simulink model "pcc_backstepping_model_unaware_full_system_PID"  (R2021b)
settings: Solver=VariableStepAuto  StartTime=0.0  StopTime=60  MaxStep=0.001  RelTol=1e-3
values from neighbouring files (symbols this model uses):
  l = out.l.Data    [animate_pcc.m]    (also in config.m = 0.110*[1;1;1])
  q_eq = [-108; 21.5; -3.4]/180*pi    [config.m]
undefined symbols (not defined in the file or in its folder): mu_p_eq, tol_q_stable
libraries: simulink_extras x4, slpidlib x1
settings Model: PauseTimes=0  Creator=maximilianstoelzle  LastModifiedBy=mstolzle
settings RTWCC: BuildConfiguration=Faster Runs

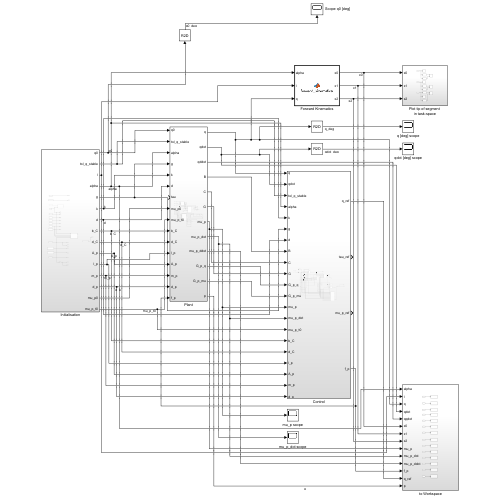
[thumbnail: Simulink's stored preview of the top-level diagram]
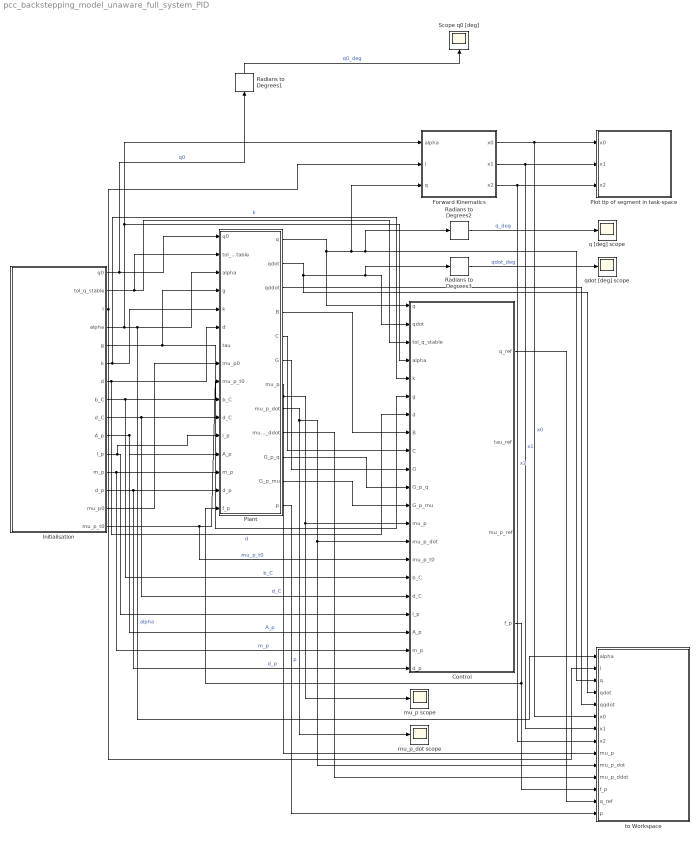
== system pcc_backstepping_model_unaware_full_system_PID ==
  Control : Subsystem
  Forward Kinematics : MATLAB Function  TreatAsAtomicUnit=on
  Initialisation : Subsystem
  Plant : Subsystem
  Plot tip of segment in task-space : Subsystem
  Radians to Degrees1 : simulink_extras/Transformations/Radians to Degrees
  Radians to Degrees2 : simulink_extras/Transformations/Radians to Degrees
  Radians to Degrees3 : simulink_extras/Transformations/Radians to Degrees
  Scope q0 [deg] : Scope
  mu_p scope : Scope
  mu_p_dot scope : Scope
  q [deg] scope : Scope
  qdot [deg] scope : Scope
  to Workspace : Subsystem
  wires:
  Plant/3(qddot) -> to Workspace/5(qqdot)
  Initialisation/12(m_p) -> Plant/14(m_p), Control/20(m_p)  "m_p"
  Initialisation/3(l) -> Forward Kinematics/2(l), to Workspace/2(l)
  Radians to Degrees2/1 -> q [deg] scope/1  "q_deg"
  Initialisation/11(l_p) -> Plant/12(l_p), Control/18(l_p)
  Initialisation/1(q0) -> Radians to Degrees1/1, Plant/1(q0)  "q0"
  Plant/9(mu_p_ddot) -> to Workspace/11(mu_p_ddot)
  Initialisation/14(mu_p0) -> Plant/8(mu_p0)
  Control/1(q_ref) -> to Workspace/13(q_ref)
  Forward Kinematics/3(x2) -> to Workspace/8(x2), Plot tip of segment in task-space/3(x2)  "x2"
  Plant/6(G) -> Control/10(G)
  Plant/11(G_p_mu) -> Control/12(G_p_mu)
  Plant/4(B) -> Control/8(B)
  Initialisation/6(k) -> Control/5(k), Plant/5(k)  "k"
  Radians to Degrees3/1 -> qdot [deg] scope/1  "qdot_deg"
  Radians to Degrees1/1 -> Scope q0 [deg]/1  "q0_deg"
  Initialisation/2(tol_q_stable) -> Plant/2(tol_q_stable), Control/3(tol_q_stable)
  Plant/10(G_p_q) -> Control/11(G_p_q)
  Plant/5(C) -> Control/9(C)
  Initialisation/13(d_p) -> Plant/15(d_p), Control/21(d_p)  "d_p"
  Initialisation/5(g) -> Plant/4(g), Control/6(g)
  Initialisation/4(alpha) -> to Workspace/1(alpha), Plant/3(alpha), Forward Kinematics/1(alpha), Control/4(alpha)  "alpha"
  Initialisation/7(d) -> Plant/6(d), Control/7(d)  "d"
  Plant/2(qdot) -> Control/2(qdot), Radians to Degrees3/1, to Workspace/4(qdot)
  Plant/1(q) -> Radians to Degrees2/1, to Workspace/3(q), Forward Kinematics/3(q), Control/1(q)
  Initialisation/10(A_p) -> Plant/13(A_p), Control/19(A_p)  "A_p"
  Initialisation/9(d_C) -> Plant/11(d_C), Control/17(d_C)  "d_C"
  Initialisation/8(b_C) -> Plant/10(b_C), Control/16(b_C)  "b_C"
  Plant/7(mu_p) -> mu_p scope/1, Control/13(mu_p), to Workspace/9(mu_p)
  Forward Kinematics/1(x0) -> to Workspace/6(x0), Plot tip of segment in task-space/1(x0)  "x0"
  Forward Kinematics/2(x1) -> to Workspace/7(x1), Plot tip of segment in task-space/2(x1)  "x1"
  Control/4(f_p) -> to Workspace/12(f_p), Plant/16(f_p)
  Plant/8(mu_p_dot) -> Control/14(mu_p_dot), to Workspace/10(mu_p_dot), mu_p_dot scope/1
  Initialisation/15(mu_p_t0) -> Control/15(mu_p_t0), Plant/9(mu_p_t0)  "mu_p_t0"
  Plant/12(p) -> to Workspace/14(p)  "p"

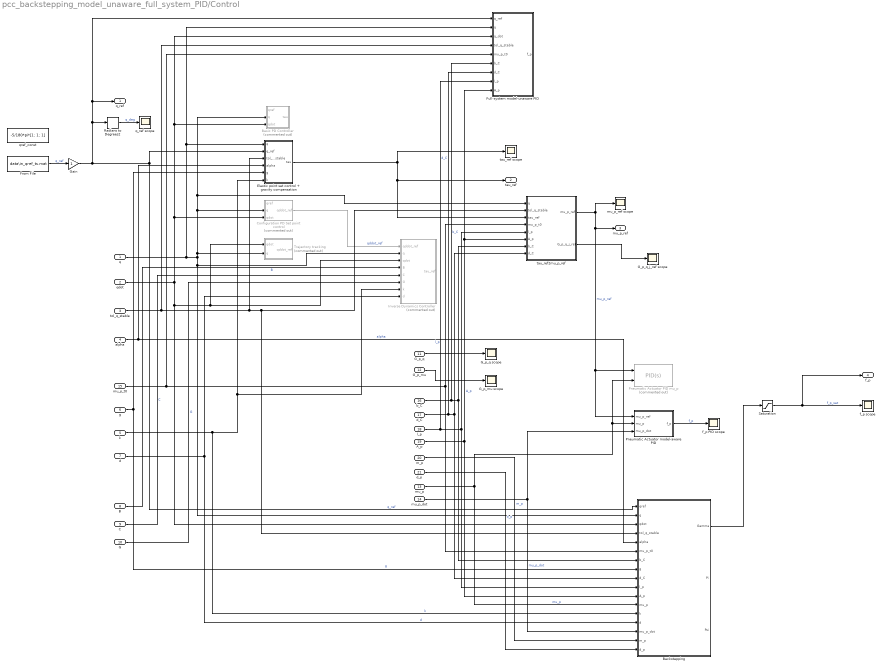
== system pcc_backstepping_model_unaware_full_system_PID/Control ==
  q : Inport
  qdot : Inport  Port=2
  tol_q_stable : Inport  Port=3
  alpha : Inport  Port=4
  k : Inport  Port=5
  g : Inport  Port=6
  d : Inport  Port=7
  B : Inport  Port=8
  C : Inport  Port=9
  G : Inport  Port=10
  G_p_q : Inport  Port=11
  G_p_mu : Inport  Port=12
  mu_p : Inport  Port=13
  mu_p_dot : Inport  Port=14
  mu_p_t0 : Inport  Port=15
  b_C : Inport  Port=16
  d_C : Inport  Port=17
  l_p : Inport  Port=18
  A_p : Inport  Port=19
  m_p : Inport  Port=20
  d_p : Inport  Port=21
  Backstepping : Subsystem
  Basic PD Controller : Subsystem  Commented=on
  Configuration PD Set point control : Subsystem  Commented=on
  Elastic point set control + gravity compensation : MATLAB Function  TreatAsAtomicUnit=on
  From File : FromFile  FileName=data\in_qref_ts.mat  SampleTime=0  InterpolationWithinTimeRange=Zero order hold
  Full-system model-unaware PID : Subsystem
  G_p_mu scope : Scope
  G_p_q scope : Scope
  G_p_q_j_ref scope : Scope
  Gain : Gain
  Inverse Dynamics Controller : MATLAB Function  Commented=on  TreatAsAtomicUnit=on
  Pneumatic Actuator PID mu_p : slpidlib/PID Controller (2DOF)  Commented=on  Controller=PID  Form=Parallel  TimeDomain=Continuous-time  UseExternalTs=off  SampleTime=-1  IntegratorMethod=Forward Euler  FilterMethod=Forward Euler  ControllerParametersSource=internal  P=-3000  I=-500  D=-100  UseFilter=on  N=100  b=1  c=1  TunerSelectOption=Frequency Response Based  InitialConditionSource=internal  InitialConditionForIntegrator=0  InitialConditionForFilter=0  DifferentiatorICPrevScaledInput=0  ExternalReset=none  TrackingMode=off  Kt=1  LimitOutput=off  SatLimitsSource=internal  UpperSaturationLimit=inf  LowerSaturationLimit=-inf  LinearizeAsGain=on  AntiWindupMode=none  Kb=1  POutMin=[]  POutMax=[]  IOutMin=[]  IOutMax=[]  DOutMin=[]  DOutMax=[]  NOutMin=[]  NOutMax=[]  bOutMin=[]  bOutMax=[]  cOutMin=[]  cOutMax=[]  SumOutMin=[]  SumOutMax=[]  SaturationOutMin=[]  SaturationOutMax=[]  PParamMin=[]  PParamMax=[]  IParamMin=[]  IParamMax=[]  DParamMin=[]  DParamMax=[]  NParamMin=[]  NParamMax=[]  bParamMin=[]  bParamMax=[]  cParamMin=[]  cParamMax=[]  KbParamMin=[]  KbParamMax=[]  KtParamMin=[]  KtParamMax=[]  KbOutMin=[]  KbOutMax=[]  KtOutMin=[]  KtOutMax=[]  IntegratorOutMin=[]  IntegratorOutMax=[]  FilterOutMin=[]  FilterOutMax=[]  SumI1OutMin=[]  SumI1OutMax=[]  SumI2OutMin=[]  SumI2OutMax=[]  SumI3OutMin=[]  SumI3OutMax=[]  SumI4OutMin=[]  SumI4OutMax=[]  SumDOutMin=[]  SumDOutMax=[]  Sum1OutMin=[]  Sum1OutMax=[]  Sum2OutMin=[]  Sum2OutMax=[]  Sum3OutMin=[]  Sum3OutMax=[]  DifferentiatorOutMin=[]  DifferentiatorOutMax=[]  FilterDiffOutCoefMin=[]  FilterDiffOutCoefMax=[]  ReciprocalOutMin=[]  ReciprocalOutMax=[]  SumDenOutMin=[]  SumDenOutMax=[]  SumNumOutMin=[]  SumNumOutMax=[]  DivideOutMin=[]  DivideOutMax=[]  UdiffTsProdOutMin=[]  UdiffTsProdOutMax=[]  NTsProdOutMin=[]  NTsProdOutMax=[]  UintegralTsProdOutMin=[]  UintegralTsProdOutMax=[]  UngainTsProdOutMin=[]  UngainTsProdOutMax=[]  IntegratorContinuousStateAttributes=''  IntegratorStateMustResolveToSignalObject=off  IntegratorRTWStateStorageClass=Auto  FilterContinuousStateAttributes=''  FilterStateMustResolveToSignalObject=off  FilterRTWStateStorageClass=Auto  ParallelPVariant=InternalParameters  IdealPVariant=Disabled  IVariant=InternalParameters  DVariant=InternalParameters  bVariant=InternalParameters  cVariant=InternalParameters  IntegratorVariant=Continuous  SatVariant=Disabled  AWVariant=Passthrough  PCopyVariant=Disabled  TRVariant=Disabled  FdbkBlocksVariant=Forward  IdealPFdbkVariant=Disabled  SatFdbkVariant=Disabled  DerivativeFilterVariant=ContFilter  NVariant=InternalParameters  NCopyVariant=Disabled  FilterICVariant=InternalICsFilter  IntegratorICVariant=InternalICs  ExternalResetVariant=Disabled  TRSumVariant=Passthrough  SumFdbkVariant=Disabled  SumVariant=Sum_PID  TsampFilterVariant=InternalTs  TsampNgainVariant=Passthrough  TsampIntegralVariant=Passthrough  ExternalSaturationOutDataTypeStr=Inherit: Same as second input
      settings: SourceProductBaseCode=SL
  Pneumatic Actuator model-aware PID : Subsystem
  Radians to Degrees2 : simulink_extras/Transformations/Radians to Degrees
  Saturation : Saturate  UpperLimit=1000  LowerLimit=-1000
  Trajectory tracking : Subsystem  Commented=on
  f_p PID scope : Scope
  f_p scope : Scope
  mu_p_ref scope : Scope
  q_ref scope : Scope
  qref_const : Constant  Value=-5/180*pi*[1; 1; 1]
  tau_ref scope : Scope
  tau_ref2mu_p_ref : MATLAB Function  TreatAsAtomicUnit=on
  q_ref : Outport
  tau_ref : Outport  Port=2
  mu_p_ref : Outport  Port=3
  f_p : Outport  Port=4
  wires:
  q/1 -> Full-system model-unaware PID/2(q), Elastic point set control + gravity compensation/1(q), Backstepping/2(q), Inverse Dynamics Controller/2(q), Trajectory tracking/2(q), Configuration PD Set point control/2(q), tau_ref2mu_p_ref/1(q), Basic PD Controller/2(q)
  qdot/1 -> Backstepping/3(qdot), Trajectory tracking/1(qdot), Inverse Dynamics Controller/3(qdot), Full-system model-unaware PID/3(q_dot), Basic PD Controller/3(qdot), Configuration PD Set point control/3(qdot)
  B/1 -> Inverse Dynamics Controller/4(B)  "B"
  C/1 -> Inverse Dynamics Controller/5(C)  "C"
  G/1 -> Inverse Dynamics Controller/6(G)  "G"
  k/1 -> Backstepping/13(k), Elastic point set control + gravity compensation/6(k), Inverse Dynamics Controller/7(k)  "k"
  d/1 -> Inverse Dynamics Controller/8(d), Backstepping/14(d)  "d"
  Configuration PD Set point control/1(qddot_ref) -> Inverse Dynamics Controller/1(qddot_ref)  "qddot_ref"
  mu_p/1 -> Pneumatic Actuator PID mu_p/2, Pneumatic Actuator model-aware PID/2(mu_p), Backstepping/12(mu_p)  "mu_p"
  tau_ref2mu_p_ref/1(mu_p_ref) -> Pneumatic Actuator model-aware PID/1(mu_p_ref), Pneumatic Actuator PID mu_p/1, mu_p_ref/1, mu_p_ref scope/1  "mu_p_ref"
  mu_p_t0/1 -> Full-system model-unaware PID/5(mu_p_t0), tau_ref2mu_p_ref/4(mu_p_t0), Backstepping/6(mu_p_t0)
  b_C/1 -> Full-system model-unaware PID/6(b_C), Backstepping/7(b_C), tau_ref2mu_p_ref/7(b_C)  "b_C"
  d_C/1 -> Full-system model-unaware PID/7(d_C), Backstepping/9(d_C), tau_ref2mu_p_ref/8(d_C)  "d_C"
  l_p/1 -> Full-system model-unaware PID/8(l_p), Backstepping/10(l_p), tau_ref2mu_p_ref/5(l_p)  "l_p"
  A_p/1 -> Full-system model-unaware PID/9(A_p), tau_ref2mu_p_ref/6(A_p), Backstepping/11(A_p)  "A_p"
  tau_ref2mu_p_ref/2(G_p_q_j_ref) -> G_p_q_j_ref scope/1
  G_p_q/1 -> G_p_q scope/1
  G_p_mu/1 -> G_p_mu scope/1
  mu_p_dot/1 -> Pneumatic Actuator model-aware PID/3(mu_p_dot), Backstepping/15(mu_p_dot)  "mu_p_dot"
  alpha/1 -> Elastic point set control + gravity compensation/4(alpha), Backstepping/5(alpha)  "alpha"
  g/1 -> Backstepping/8(g), Elastic point set control + gravity compensation/5(g)  "g"
  Elastic point set control + gravity compensation/1(tau) -> tau_ref/1, tau_ref2mu_p_ref/3(tau_ref), tau_ref scope/1
  Saturation/1 -> f_p/1, f_p scope/1  "f_p_sat"
  m_p/1 -> Backstepping/16(m_p)  "m_p"
  Gain/1 -> Full-system model-unaware PID/1(q_ref), q_ref/1, Radians to Degrees2/1, Backstepping/1(qref), Elastic point set control + gravity compensation/2(q_ref)  "q_ref"
  From File/1 -> Gain/1  "q_ref"
  tol_q_stable/1 -> Full-system model-unaware PID/4(tol_q_stable), Elastic point set control + gravity compensation/3(tol_q_stable), Backstepping/4(tol_q_stable), tau_ref2mu_p_ref/2(tol_q_stable)
  Radians to Degrees2/1 -> q_ref scope/1  "q_deg"
  d_p/1 -> Backstepping/17(d_p)  "d_p"
  Pneumatic Actuator model-aware PID/1(f_p) -> f_p PID scope/1  "f_p"
  Backstepping/1(Gamma) -> Saturation/1

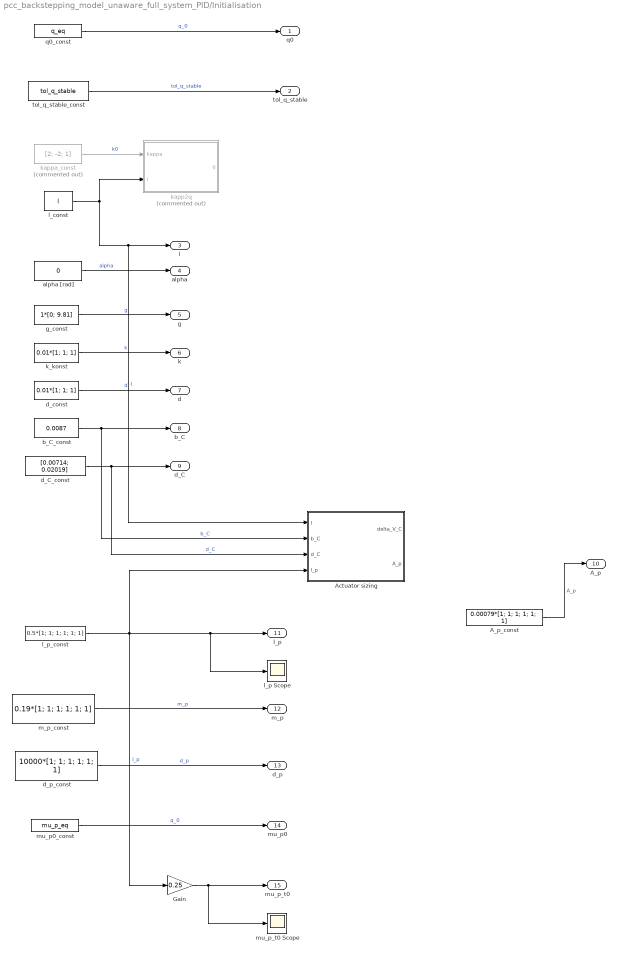
== system pcc_backstepping_model_unaware_full_system_PID/Initialisation ==
  A_p_const : Constant  Value=0.00079*[1; 1; 1; 1; 1; 1]
  Actuator sizing : MATLAB Function  TreatAsAtomicUnit=on
  Gain : Gain  Gain=0.25
  alpha [rad] : Constant  Value=0
  b_C_const : Constant  Value=0.0087
  d_C_const : Constant  Value=[0.00714; 0.02019]
  d_const : Constant  Value=0.01*[1; 1; 1]
  d_p_const : Constant  Value=10000*[1; 1; 1; 1; 1; 1]
  g_const : Constant  Value=1*[0; 9.81]
  k_konst : Constant  Value=0.01*[1; 1; 1]
  kapp2q : MATLAB Function  Commented=on  TreatAsAtomicUnit=on
  kappa_const : Constant  Commented=on  Value=[2; -2; 1]
  l_const : Constant  Value=l
  l_p Scope : Scope
  l_p_const : Constant  Value=0.5*[1; 1; 1; 1; 1; 1]
  m_p_const : Constant  Value=0.19*[1; 1; 1; 1; 1; 1]
  mu_p0_const : Constant  Value=mu_p_eq
  mu_p_t0 Scope : Scope
  q0_const : Constant  Value=q_eq
  tol_q_stable_const : Constant  Value=tol_q_stable
  q0 : Outport
  tol_q_stable : Outport  Port=2
  l : Outport  Port=3
  alpha : Outport  Port=4
  g : Outport  Port=5
  k : Outport  Port=6
  d : Outport  Port=7
  b_C : Outport  Port=8
  d_C : Outport  Port=9
  A_p : Outport  Port=10
  l_p : Outport  Port=11
  m_p : Outport  Port=12
  d_p : Outport  Port=13
  mu_p0 : Outport  Port=14
  mu_p_t0 : Outport  Port=15
  wires:
  kappa_const/1 -> kapp2q/1(kappa)  "k0"
  l_const/1 -> Actuator sizing/1(l), l/1, kapp2q/2(l)  "l"
  alpha [rad]/1 -> alpha/1  "alpha"
  g_const/1 -> g/1  "g"
  k_konst/1 -> k/1  "k"
  d_C_const/1 -> Actuator sizing/3(d_C), d_C/1  "d_C"
  m_p_const/1 -> m_p/1  "m_p"
  b_C_const/1 -> Actuator sizing/2(b_C), b_C/1  "b_C"
  l_p_const/1 -> Gain/1, Actuator sizing/4(l_p), l_p Scope/1, l_p/1  "l_p"
  Gain/1 -> mu_p_t0 Scope/1, mu_p_t0/1
  d_const/1 -> d/1  "d"
  A_p_const/1 -> A_p/1  "A_p"
  q0_const/1 -> q0/1  "q_0"
  tol_q_stable_const/1 -> tol_q_stable/1  "tol_q_stable"
  mu_p0_const/1 -> mu_p0/1  "q_0"
  d_p_const/1 -> d_p/1  "d_p"

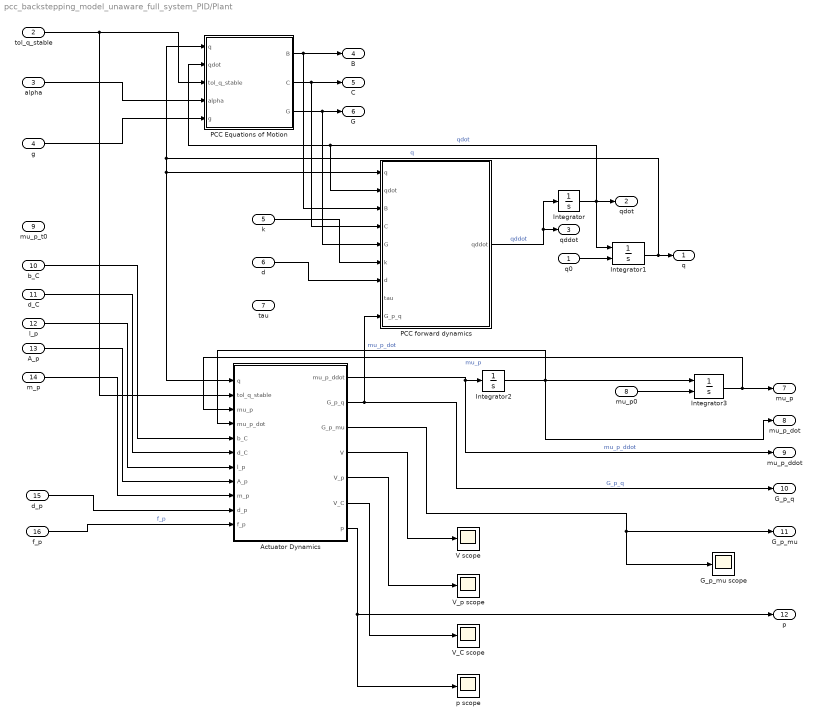
== system pcc_backstepping_model_unaware_full_system_PID/Plant ==
  q0 : Inport
  tol_q_stable : Inport  Port=2
  alpha : Inport  Port=3
  g : Inport  Port=4
  k : Inport  Port=5
  d : Inport  Port=6
  tau : Inport  Port=7
  mu_p0 : Inport  Port=8
  mu_p_t0 : Inport  Port=9
  b_C : Inport  Port=10
  d_C : Inport  Port=11
  l_p : Inport  Port=12
  A_p : Inport  Port=13
  m_p : Inport  Port=14
  d_p : Inport  Port=15
  f_p : Inport  Port=16
  Actuator Dynamics : MATLAB Function  TreatAsAtomicUnit=on
  G_p_mu scope : Scope
  Integrator : Integrator  InitialCondition=[0; 0; 0]
  Integrator1 : Integrator  InitialConditionSource=external
  Integrator2 : Integrator  InitialCondition=[0; 0; 0; 0; 0; 0]
  Integrator3 : Integrator  InitialConditionSource=external  LowerSaturationLimit=[0; 0; 0; 0; 0; 0]
  PCC Equations of Motion : MATLAB Function  TreatAsAtomicUnit=on
  PCC forward dynamics : MATLAB Function  TreatAsAtomicUnit=on
  V scope : Scope
  V_C scope : Scope
  V_p scope : Scope
  p scope : Scope
  q : Outport
  qdot : Outport  Port=2
  qddot : Outport  Port=3
  B : Outport  Port=4
  C : Outport  Port=5
  G : Outport  Port=6
  mu_p : Outport  Port=7
  mu_p_dot : Outport  Port=8
  mu_p_ddot : Outport  Port=9
  G_p_q : Outport  Port=10
  G_p_mu : Outport  Port=11
  p : Outport  Port=12
  wires:
  g/1 -> PCC Equations of Motion/5(g)
  alpha/1 -> PCC Equations of Motion/4(alpha)
  q0/1 -> Integrator1/2
  k/1 -> PCC forward dynamics/6(k)
  PCC Equations of Motion/3(G) -> PCC forward dynamics/5(G), G/1
  PCC Equations of Motion/1(B) -> PCC forward dynamics/3(B), B/1
  Integrator1/1 -> PCC Equations of Motion/1(q), PCC forward dynamics/1(q), Actuator Dynamics/1(q), q/1  "q"
  PCC forward dynamics/1(qddot) -> Integrator/1, qddot/1  "qddot"
  d/1 -> PCC forward dynamics/7(d)
  Integrator/1 -> PCC forward dynamics/2(qdot), PCC Equations of Motion/2(qdot), Integrator1/1, qdot/1  "qdot"
  PCC Equations of Motion/2(C) -> PCC forward dynamics/4(C), C/1
  A_p/1 -> Actuator Dynamics/8(A_p)
  m_p/1 -> Actuator Dynamics/9(m_p)
  Actuator Dynamics/1(mu_p_ddot) -> mu_p_ddot/1, Integrator2/1  "mu_p_ddot"
  d_C/1 -> Actuator Dynamics/6(d_C)
  Integrator2/1 -> Actuator Dynamics/4(mu_p_dot), mu_p_dot/1, Integrator3/1  "mu_p_dot"
  b_C/1 -> Actuator Dynamics/5(b_C)
  l_p/1 -> Actuator Dynamics/7(l_p)
  Integrator3/1 -> Actuator Dynamics/3(mu_p), mu_p/1  "mu_p"
  Actuator Dynamics/2(G_p_q) -> PCC forward dynamics/9(G_p_q), G_p_q/1  "G_p_q"
  Actuator Dynamics/3(G_p_mu) -> G_p_mu scope/1, G_p_mu/1
  f_p/1 -> Actuator Dynamics/11(f_p)  "f_p"
  Actuator Dynamics/4(V) -> V scope/1
  Actuator Dynamics/6(V_C) -> V_C scope/1
  Actuator Dynamics/5(V_p) -> V_p scope/1
  tol_q_stable/1 -> Actuator Dynamics/2(tol_q_stable), PCC Equations of Motion/3(tol_q_stable)
  mu_p0/1 -> Integrator3/2
  d_p/1 -> Actuator Dynamics/10(d_p)
  Actuator Dynamics/7(p) -> p/1, p scope/1

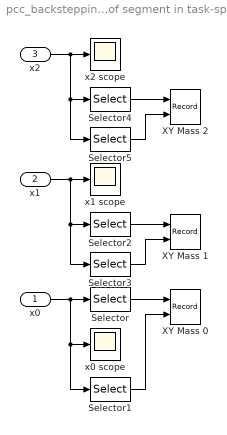
== system pcc_backstepping_model_unaware_full_system_PID/Plot tip of segment in task-space ==
  x0 : Inport
  x1 : Inport  Port=2
  x2 : Inport  Port=3
  Selector : Selector  InputPortWidth=2  IndexOptions=Index vector (dialog)  Indices=[1]  OutputSizes=1
  Selector1 : Selector  InputPortWidth=2  IndexOptions=Index vector (dialog)  Indices=[2]  OutputSizes=1
  Selector2 : Selector  InputPortWidth=2  IndexOptions=Index vector (dialog)  Indices=[1]  OutputSizes=1
  Selector3 : Selector  InputPortWidth=2  IndexOptions=Index vector (dialog)  Indices=[2]  OutputSizes=1
  Selector4 : Selector  InputPortWidth=2  IndexOptions=Index vector (dialog)  Indices=[1]  OutputSizes=1
  Selector5 : Selector  InputPortWidth=2  IndexOptions=Index vector (dialog)  Indices=[2]  OutputSizes=1
  XY Mass 0 : Record  FileSettingsInternal="{\"entries\":[{\"content\":{\"excelSettings\":{\"content\":{},\"type\":\"Streamout.ExcelSettings\"}},\"type\":\"Streamout.FileSettingStorage\",\"uuid\":\"2c9bfc5a-c848-44e7-aeaf-cc9cdd5e0af6\"}],\"packageUris\":[\"http://schema.mathworks.com/mf0/streamout_blocks/R2020a\"],\"version\":\"1.0\"}"  Layout=[1 1]  SignalsInternal="{\"entries\":[{\"content\":{\"signals\":[{\"content\":{\"blockPath\":[\"pcc_backstepping_model_unaware_full_system_PID/Plot tip of segment  in task-space/XY Mass 0\"],\"channel\":[],\"dimensions\":[1],\"domain\":\"pcc_backstepping_model_unaware_full_system_PID/Plot tip of segment  in task-space/XY Mass 0\",\"lineColor\":\"#a2142f\",\"plots\":[1],\"port\":1,\"sid\":[\"\"],\"signalID\":586916,\"signalName\":\"Selector\"},\"type\":\"RecordBlkView.Signal\",\"uuid\":\"a03f31b1-010c-4470-bf0c-6071344e1f42\"},{\"content\":{\"blockPath\":[\"pcc_backstepping_model_unaware_full_system_PID/Plot tip of segment  in task-space/XY Mass 0\"],\"channel\":[],\"dimensions\":[1],\"domain\":\"pcc_backstepping_model_unaware_full_system_PID/Plot tip of segment  in task-space/XY Mass 0\",\"lineColor\":\"#139fff\",\"plots\":[1],\"port\":2,\"sid\":[\"\"],\"signalID\":586920,\"signalName\":\"Selector1\"},\"type\":\"RecordBlkView.Signal\",\"uuid\":\"fb98b674-d954-431b-8400-e1634dfae15b\"}]},\"type\":\"RecordBlkView.InputSignals\",\"uuid\":\"48c4a9c1-d538-4b06-bec8-5126b0e2cae4\"}],\"packageUris\":[\"http://schema.mathworks.com/mf0/streamout_blocks/R2020a\"],\"version\":\"1.0\"}"  VisualizationBindings="{\"xyplotplugin\":{\"info\":[{\"series\":[{\"bindingParametersList\":[{\"parameter\":\"X-Axis\",\"signalID\":586916,\"signalName\":\"Selector\"},{\"parameter\":\"Y-Axis\",\"signalID\":586920,\"signalName\":\"Selector1\"}],\"seriesID\":59992}],\"subplotID\":1}]}}"  CompatibilityTag=XY  st=-1
  XY Mass 1 : Record  FileSettingsInternal="{\"entries\":[{\"content\":{\"excelSettings\":{\"content\":{},\"type\":\"Streamout.ExcelSettings\"}},\"type\":\"Streamout.FileSettingStorage\",\"uuid\":\"39a9d6ad-33ff-41f6-a3f9-cd83a5805264\"}],\"packageUris\":[\"http://schema.mathworks.com/mf0/streamout_blocks/R2020a\"],\"version\":\"1.0\"}"  Layout=[1 1]  SignalsInternal="{\"entries\":[{\"content\":{\"signals\":[{\"content\":{\"blockPath\":[\"pcc_backstepping_model_unaware_full_system_PID/Plot tip of segment  in task-space/XY Mass 1\"],\"channel\":[],\"dimensions\":[1],\"domain\":\"pcc_backstepping_model_unaware_full_system_PID/Plot tip of segment  in task-space/XY Mass 1\",\"lineColor\":\"#a2142f\",\"plots\":[1],\"port\":1,\"sid\":[\"\"],\"signalID\":586924,\"signalName\":\"Selector2\"},\"type\":\"RecordBlkView.Signal\",\"uuid\":\"48cd44ef-b686-4984-949c-8ea4778ecd4f\"},{\"content\":{\"blockPath\":[\"pcc_backstepping_model_unaware_full_system_PID/Plot tip of segment  in task-space/XY Mass 1\"],\"channel\":[],\"dimensions\":[1],\"domain\":\"pcc_backstepping_model_unaware_full_system_PID/Plot tip of segment  in task-space/XY Mass 1\",\"lineColor\":\"#139fff\",\"plots\":[1],\"port\":2,\"sid\":[\"\"],\"signalID\":586928,\"signalName\":\"Selector3\"},\"type\":\"RecordBlkView.Signal\",\"uuid\":\"19891226-1979-4de8-952c-68241f8af5f5\"}]},\"type\":\"RecordBlkView.InputSignals\",\"uuid\":\"71f4fa0a-7eb9-4c2a-9fa7-41728afc1426\"}],\"packageUris\":[\"http://schema.mathworks.com/mf0/streamout_blocks/R2020a\"],\"version\":\"1.0\"}"  VisualizationBindings="{\"xyplotplugin\":{\"info\":[{\"series\":[{\"bindingParametersList\":[{\"parameter\":\"X-Axis\",\"signalID\":586924,\"signalName\":\"Selector2\"},{\"parameter\":\"Y-Axis\",\"signalID\":586928,\"signalName\":\"Selector3\"}],\"seriesID\":8309}],\"subplotID\":1}]}}"  CompatibilityTag=XY  st=-1
  XY Mass 2 : Record  FileSettingsInternal="{\"entries\":[{\"content\":{\"excelSettings\":{\"content\":{},\"type\":\"Streamout.ExcelSettings\"}},\"type\":\"Streamout.FileSettingStorage\",\"uuid\":\"6f9f4c64-d47a-4205-8187-0ec534d51e43\"}],\"packageUris\":[\"http://schema.mathworks.com/mf0/streamout_blocks/R2020a\"],\"version\":\"1.0\"}"  Layout=[1 1]  SignalsInternal="{\"entries\":[{\"content\":{\"signals\":[{\"content\":{\"blockPath\":[\"pcc_backstepping_model_unaware_full_system_PID/Plot tip of segment  in task-space/XY Mass 2\"],\"channel\":[],\"dimensions\":[1],\"domain\":\"pcc_backstepping_model_unaware_full_system_PID/Plot tip of segment  in task-space/XY Mass 2\",\"lineColor\":\"#a2142f\",\"plots\":[1],\"port\":1,\"sid\":[\"\"],\"signalID\":586932,\"signalName\":\"Selector4\"},\"type\":\"RecordBlkView.Signal\",\"uuid\":\"e16da4ae-c0f3-4bd1-9ef1-f1fd4f3216e7\"},{\"content\":{\"blockPath\":[\"pcc_backstepping_model_unaware_full_system_PID/Plot tip of segment  in task-space/XY Mass 2\"],\"channel\":[],\"dimensions\":[1],\"domain\":\"pcc_backstepping_model_unaware_full_system_PID/Plot tip of segment  in task-space/XY Mass 2\",\"lineColor\":\"#139fff\",\"plots\":[1],\"port\":2,\"sid\":[\"\"],\"signalID\":586936,\"signalName\":\"Selector5\"},\"type\":\"RecordBlkView.Signal\",\"uuid\":\"8f4e5351-45a0-4f9a-9e77-fec6d654b4b2\"}]},\"type\":\"RecordBlkView.InputSignals\",\"uuid\":\"48fa3bb8-beee-4ce6-b1fb-c7d9023a848c\"}],\"packageUris\":[\"http://schema.mathworks.com/mf0/streamout_blocks/R2020a\"],\"version\":\"1.0\"}"  VisualizationBindings="{\"xyplotplugin\":{\"info\":[{\"series\":[{\"bindingParametersList\":[{\"parameter\":\"X-Axis\",\"signalID\":586932,\"signalName\":\"Selector4\"},{\"parameter\":\"Y-Axis\",\"signalID\":586936,\"signalName\":\"Selector5\"}],\"seriesID\":15249}],\"subplotID\":1}]}}"  CompatibilityTag=XY  st=-1
  x0 scope : Scope
  x1 scope : Scope
  x2 scope : Scope
  wires:
  x2/1 -> Selector5/1, Selector4/1, x2 scope/1
  Selector/1 -> XY Mass 0/1
  x1/1 -> Selector3/1, Selector2/1, x1 scope/1
  Selector5/1 -> XY Mass 2/2
  Selector3/1 -> XY Mass 1/2
  Selector1/1 -> XY Mass 0/2
  x0/1 -> x0 scope/1, Selector1/1, Selector/1
  Selector4/1 -> XY Mass 2/1
  Selector2/1 -> XY Mass 1/1

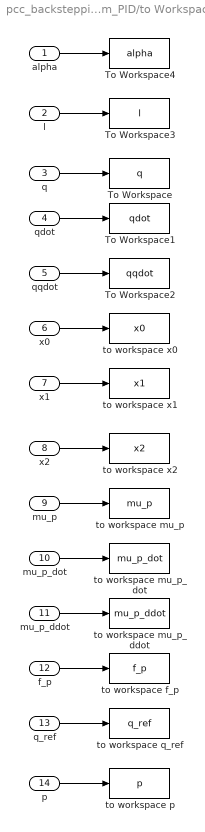
== system pcc_backstepping_model_unaware_full_system_PID/to Workspace ==
  alpha : Inport
  l : Inport  Port=2
  q : Inport  Port=3
  qdot : Inport  Port=4
  qqdot : Inport  Port=5
  x0 : Inport  Port=6
  x1 : Inport  Port=7
  x2 : Inport  Port=8
  mu_p : Inport  Port=9
  mu_p_dot : Inport  Port=10
  mu_p_ddot : Inport  Port=11
  f_p : Inport  Port=12
  q_ref : Inport  Port=13
  p : Inport  Port=14
  To Workspace : ToWorkspace  VariableName=q  SaveFormat=Timeseries  SampleTime=-1
  To Workspace1 : ToWorkspace  VariableName=qdot  SaveFormat=Timeseries  SampleTime=-1
  To Workspace2 : ToWorkspace  VariableName=qqdot  SaveFormat=Timeseries  SampleTime=-1
  To Workspace3 : ToWorkspace  VariableName=l  SaveFormat=Timeseries  SampleTime=-1
  To Workspace4 : ToWorkspace  VariableName=alpha  SaveFormat=Timeseries  SampleTime=-1
  to workspace f_p : ToWorkspace  VariableName=f_p  SaveFormat=Timeseries  SampleTime=-1
  to workspace mu_p : ToWorkspace  VariableName=mu_p  SaveFormat=Timeseries  SampleTime=-1
  to workspace mu_p_ddot : ToWorkspace  VariableName=mu_p_ddot  SaveFormat=Timeseries  SampleTime=-1
  to workspace mu_p_dot : ToWorkspace  VariableName=mu_p_dot  SaveFormat=Timeseries  SampleTime=-1
  to workspace p : ToWorkspace  VariableName=p  SaveFormat=Timeseries  SampleTime=-1
  to workspace q_ref : ToWorkspace  VariableName=q_ref  SaveFormat=Timeseries  SampleTime=-1
  to workspace x0 : ToWorkspace  VariableName=x0  SaveFormat=Timeseries  SampleTime=-1
  to workspace x1 : ToWorkspace  VariableName=x1  SaveFormat=Timeseries  SampleTime=-1
  to workspace x2 : ToWorkspace  VariableName=x2  SaveFormat=Timeseries  SampleTime=-1
  wires:
  alpha/1 -> To Workspace4/1
  qdot/1 -> To Workspace1/1
  l/1 -> To Workspace3/1
  qqdot/1 -> To Workspace2/1
  q/1 -> To Workspace/1
  mu_p/1 -> to workspace mu_p/1
  mu_p_dot/1 -> to workspace mu_p_dot/1
  mu_p_ddot/1 -> to workspace mu_p_ddot/1
  f_p/1 -> to workspace f_p/1
  q_ref/1 -> to workspace q_ref/1
  x0/1 -> to workspace x0/1
  x1/1 -> to workspace x1/1
  x2/1 -> to workspace x2/1
  p/1 -> to workspace p/1

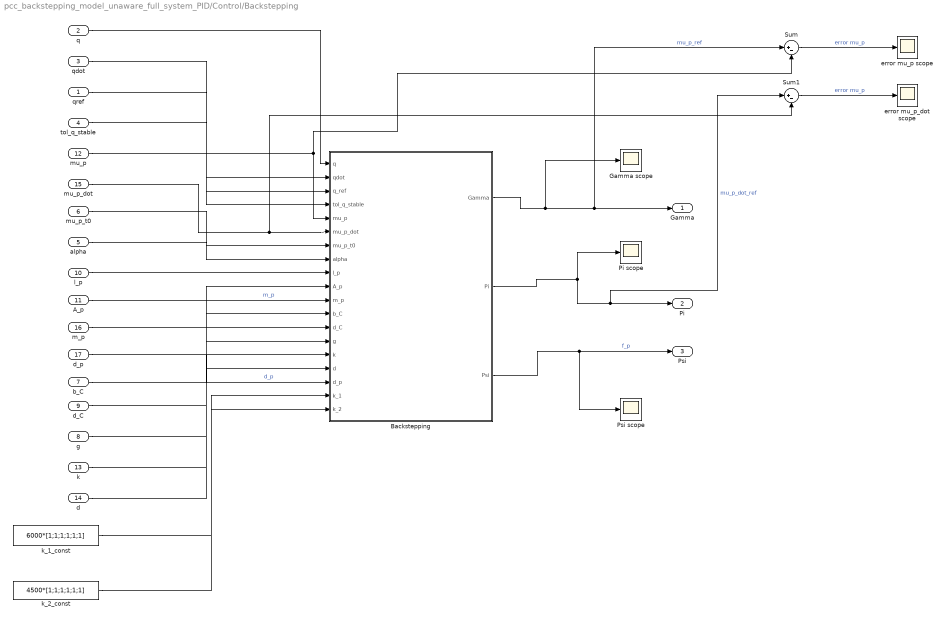
== system pcc_backstepping_model_unaware_full_system_PID/Control/Backstepping ==
  qref : Inport
  q : Inport  Port=2
  qdot : Inport  Port=3
  tol_q_stable : Inport  Port=4
  alpha : Inport  Port=5
  mu_p_t0 : Inport  Port=6
  b_C : Inport  Port=7
  g : Inport  Port=8
  d_C : Inport  Port=9
  l_p : Inport  Port=10
  A_p : Inport  Port=11
  mu_p : Inport  Port=12
  k : Inport  Port=13
  d : Inport  Port=14
  mu_p_dot : Inport  Port=15
  m_p : Inport  Port=16
  d_p : Inport  Port=17
  Backstepping : MATLAB Function  TreatAsAtomicUnit=on
  Gamma scope : Scope
  Pi scope : Scope
  Psi scope : Scope
  Sum : Sum  Inputs=|+-
  Sum1 : Sum  Inputs=|+-
  error mu_p scope : Scope
  error mu_p_dot scope : Scope
  k_1_const : Constant  Value=6000*[1;1;1;1;1;1]
  k_2_const : Constant  Value=4500*[1;1;1;1;1;1]
  Gamma : Outport
  Pi : Outport  Port=2
  Psi : Outport  Port=3
  wires:
  k_2_const/1 -> Backstepping/19(k_2)
  mu_p/1 -> Backstepping/5(mu_p), Sum/2
  k_1_const/1 -> Backstepping/18(k_1)
  qref/1 -> Backstepping/3(q_ref)
  q/1 -> Backstepping/1(q)
  Backstepping/2(Pi) -> Sum1/1, Pi/1, Pi scope/1  "mu_p_dot_ref"
  Backstepping/1(Gamma) -> Sum/1, Gamma/1, Gamma scope/1  "mu_p_ref"
  qdot/1 -> Backstepping/2(qdot)
  A_p/1 -> Backstepping/10(A_p)
  k/1 -> Backstepping/15(k)
  alpha/1 -> Backstepping/8(alpha)
  mu_p_dot/1 -> Sum1/2, Backstepping/6(mu_p_dot)
  b_C/1 -> Backstepping/12(b_C)
  d_C/1 -> Backstepping/13(d_C)
  g/1 -> Backstepping/14(g)
  d/1 -> Backstepping/16(d)
  l_p/1 -> Backstepping/9(l_p)
  mu_p_t0/1 -> Backstepping/7(mu_p_t0)
  Backstepping/3(Psi) -> Psi/1, Psi scope/1  "f_p"
  Sum/1 -> error mu_p scope/1  "error mu_p"
  Sum1/1 -> error mu_p_dot scope/1  "error mu_p"
  m_p/1 -> Backstepping/11(m_p)  "m_p"
  tol_q_stable/1 -> Backstepping/4(tol_q_stable)
  d_p/1 -> Backstepping/17(d_p)  "d_p"

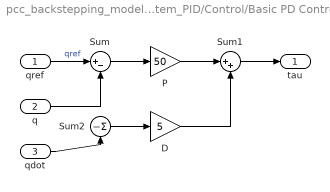
== system pcc_backstepping_model_unaware_full_system_PID/Control/Basic PD Controller ==
  qref : Inport
  q : Inport  Port=2
  qdot : Inport  Port=3
  D : Gain  Gain=5
  P : Gain  Gain=50
  Sum : Sum  Inputs=|+-
  Sum1 : Sum  Inputs=|++
  Sum2 : Sum  Inputs=||-
  tau : Outport
  wires:
  qdot/1 -> Sum2/1
  Sum1/1 -> tau/1
  D/1 -> Sum1/2
  q/1 -> Sum/2
  qref/1 -> Sum/1  "qref"
  Sum/1 -> P/1
  P/1 -> Sum1/1
  Sum2/1 -> D/1

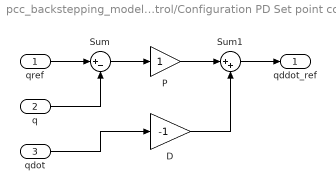
== system pcc_backstepping_model_unaware_full_system_PID/Control/Configuration PD Set point control ==
  qref : Inport
  q : Inport  Port=2
  qdot : Inport  Port=3
  D : Gain  Gain=-1
  P : Gain
  Sum : Sum  Inputs=|+-
  Sum1 : Sum  Inputs=|++
  qddot_ref : Outport
  wires:
  Sum1/1 -> qddot_ref/1
  D/1 -> Sum1/2
  q/1 -> Sum/2
  qref/1 -> Sum/1
  Sum/1 -> P/1
  P/1 -> Sum1/1
  qdot/1 -> D/1

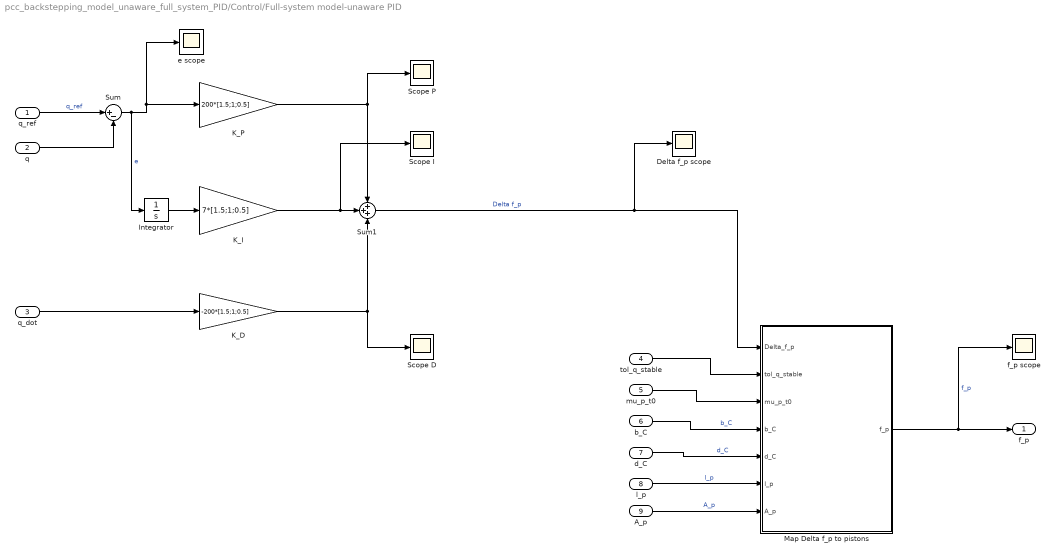
== system pcc_backstepping_model_unaware_full_system_PID/Control/Full-system model-unaware PID ==
  q_ref : Inport
  q : Inport  Port=2
  q_dot : Inport  Port=3
  tol_q_stable : Inport  Port=4
  mu_p_t0 : Inport  Port=5
  b_C : Inport  Port=6
  d_C : Inport  Port=7
  l_p : Inport  Port=8
  A_p : Inport  Port=9
  Delta f_p scope : Scope
  Integrator : Integrator
  K_D : Gain  Gain=-200*[1.5;1;0.5]
  K_I : Gain  Gain=7*[1.5;1;0.5]
  K_P : Gain  Gain=200*[1.5;1;0.5]
  Map Delta f_p to pistons : MATLAB Function  TreatAsAtomicUnit=on
  Scope D : Scope
  Scope I : Scope
  Scope P : Scope
  Sum : Sum  Inputs=|+-
  Sum1 : Sum  Inputs=+++
  e scope : Scope
  f_p scope : Scope
  f_p : Outport
  wires:
  K_D/1 -> Sum1/3, Scope D/1
  q/1 -> Sum/2
  q_ref/1 -> Sum/1  "q_ref"
  Sum/1 -> e scope/1, K_P/1, Integrator/1  "e"
  K_P/1 -> Scope P/1, Sum1/1
  q_dot/1 -> K_D/1
  Integrator/1 -> K_I/1
  K_I/1 -> Scope I/1, Sum1/2
  Sum1/1 -> Delta f_p scope/1, Map Delta f_p to pistons/1(Delta_f_p)  "Delta f_p"
  Map Delta f_p to pistons/1(f_p) -> f_p scope/1, f_p/1  "f_p"
  mu_p_t0/1 -> Map Delta f_p to pistons/3(mu_p_t0)
  d_C/1 -> Map Delta f_p to pistons/5(d_C)  "d_C"
  b_C/1 -> Map Delta f_p to pistons/4(b_C)  "b_C"
  l_p/1 -> Map Delta f_p to pistons/6(l_p)  "l_p"
  A_p/1 -> Map Delta f_p to pistons/7(A_p)  "A_p"
  tol_q_stable/1 -> Map Delta f_p to pistons/2(tol_q_stable)

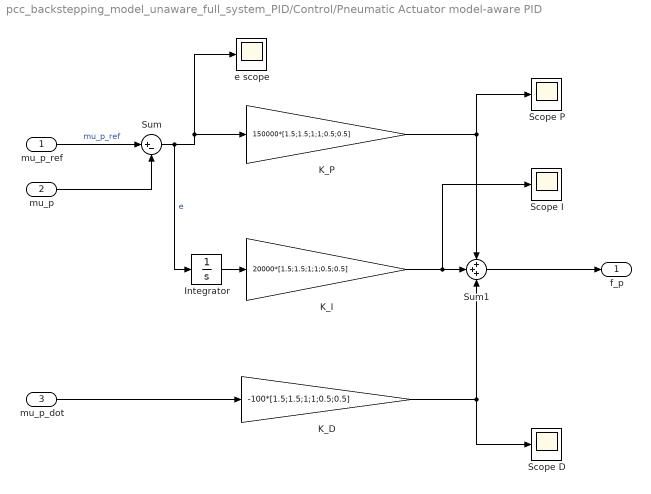
== system pcc_backstepping_model_unaware_full_system_PID/Control/Pneumatic Actuator model-aware PID ==
  mu_p_ref : Inport
  mu_p : Inport  Port=2
  mu_p_dot : Inport  Port=3
  Integrator : Integrator
  K_D : Gain  Gain=-100*[1.5;1.5;1;1;0.5;0.5]
  K_I : Gain  Gain=20000*[1.5;1.5;1;1;0.5;0.5]
  K_P : Gain  Gain=150000*[1.5;1.5;1;1;0.5;0.5]
  Scope D : Scope
  Scope I : Scope
  Scope P : Scope
  Sum : Sum  Inputs=|+-
  Sum1 : Sum  Inputs=+++
  e scope : Scope
  f_p : Outport
  wires:
  Sum1/1 -> f_p/1
  K_D/1 -> Sum1/3, Scope D/1
  mu_p/1 -> Sum/2
  mu_p_ref/1 -> Sum/1  "mu_p_ref"
  Sum/1 -> e scope/1, K_P/1, Integrator/1  "e"
  K_P/1 -> Scope P/1, Sum1/1
  mu_p_dot/1 -> K_D/1
  Integrator/1 -> K_I/1
  K_I/1 -> Scope I/1, Sum1/2

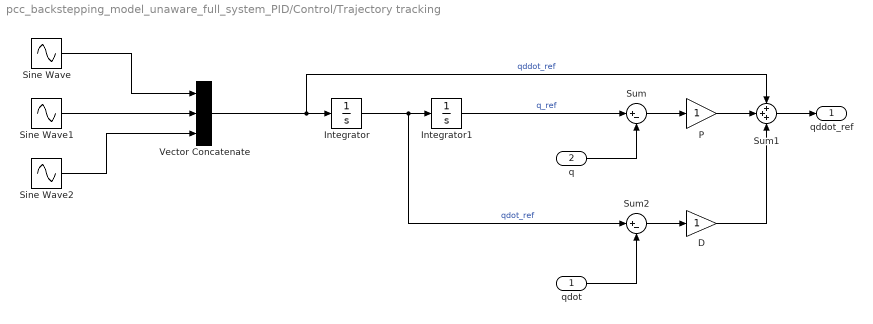
== system pcc_backstepping_model_unaware_full_system_PID/Control/Trajectory tracking ==
  qdot : Inport
  q : Inport  Port=2
  D : Gain
  Integrator : Integrator  InitialCondition=[-0.25, -0.5, -1]
  Integrator1 : Integrator
  P : Gain
  Sine Wave : Sin  Amplitude=0.25  Samples=100  SampleTime=0
  Sine Wave1 : Sin  Amplitude=0.5  SampleTime=0
  Sine Wave2 : Sin  SampleTime=0
  Sum : Sum  Inputs=|+-
  Sum1 : Sum  Inputs=+++
  Sum2 : Sum  Inputs=|+-
  Vector Concatenate : Concatenate  NumInputs=3
  qddot_ref : Outport
  wires:
  Sum1/1 -> qddot_ref/1
  q/1 -> Sum/2
  Sum/1 -> P/1
  Vector Concatenate/1 -> Sum1/1, Integrator/1  "qddot_ref"
  Integrator/1 -> Sum2/1, Integrator1/1  "qdot_ref"
  Integrator1/1 -> Sum/1  "q_ref"
  qdot/1 -> Sum2/2
  Sum2/1 -> D/1
  D/1 -> Sum1/3
  P/1 -> Sum1/2
  Sine Wave/1 -> Vector Concatenate/1
  Sine Wave1/1 -> Vector Concatenate/2
  Sine Wave2/1 -> Vector Concatenate/3

== matlab function pcc_backstepping_model_unaware_full_system_PID/Control/Elastic point set control + gravity compensation ==
  data: q input; q_ref input; tol_q_stable input; alpha input; g input; tau output; k input
function tau = fcn(q, q_ref, tol_q_stable, alpha, g, k)
    % introduce tolerance for numerical stability
    q_stable = set_min_abs_val(q, tol_q_stable);
    % q_ref_stable = set_min_abs_val(q_ref, tol_q_stable);
    
    G = G_fun(q_stable, alpha, g);
    % G_ref = G_fun(q_ref_stable, alpha, g);

    tau = k.*q_ref + G;
end

== matlab function pcc_backstepping_model_unaware_full_system_PID/Plant/Actuator Dynamics ==
  data: mu_p_ddot output; q input; tol_q_stable input; mu_p input; mu_p_dot input; b_C input; d_C input; l_p input; A_p input; G_p_q output; G_p_mu output; m_p input; d_p input; f_p input; V output; V_p output; V_C output; p output
function [mu_p_ddot, G_p_q, G_p_mu, V, V_p, V_C, p]  = actuator_dynamics(q, tol_q_stable, mu_p, mu_p_dot, b_C, d_C, l_p, A_p, m_p, d_p, f_p)
    % introduce tolerance for numerical stability
    q_stable = set_min_abs_val(q, tol_q_stable);

    % volume of fluid
    V = V_fun(q_stable, mu_p, A_p, b_C, d_C);
    V_p = V_p_fun(mu_p, A_p);
    V_C = V_C_fun(q_stable, b_C, d_C);

    % pressure in the system
    p = p_fun(q, mu_p, l_p, A_p, b_C, d_C);

    % potential forces by fluid
    G_p_q = G_p_q_fun(q_stable, mu_p, l_p, A_p, b_C, d_C);
    G_p_mu = G_p_mu_fun(q_stable, mu_p, l_p, A_p, b_C, d_C);
    
    M_p = diag(m_p);
    
    mu_p_ddot = M_p^(-1)*(f_p-G_p_mu-d_p.*mu_p_dot);
end

== matlab function pcc_backstepping_model_unaware_full_system_PID/Initialisation/Actuator sizing ==
  data: l input; delta_V_C output; b_C input; d_C input; l_p input; A_p output
function [delta_V_C, A_p]= piston_sizing(l, b_C, d_C, l_p)
    q_min = -90/180*pi*ones(length(l), 1);
    q_max = 90/180*pi*ones(length(l), 1);
    delta_V_C = abs(V_C_fun(q_max, b_C, d_C) - V_C_fun(q_min, b_C, d_C));
    A_p = 1*delta_V_C ./ l_p;
end

== matlab function pcc_backstepping_model_unaware_full_system_PID/Control/tau_ref2mu_p_ref ==
  data: q input; tol_q_stable input; tau_ref input; mu_p_ref output; mu_p_t0 input; l_p input; A_p input; b_C input; d_C input; G_p_q_j_ref output
function [mu_p_ref, G_p_q_j_ref]= tau_ref2mu_p_ref(q, tol_q_stable, tau_ref, mu_p_t0, l_p, A_p, b_C, d_C)
    % introduce tolerance for numerical stability
    q_stable = set_min_abs_val(q, tol_q_stable);

    mu_p_ref = mu_p_ref_fun(q_stable, tau_ref, mu_p_t0, l_p, A_p, b_C, d_C);
    G_p_q_j_ref = G_p_q_j_ref_fun(tau_ref, mu_p_t0, l_p, A_p, b_C, d_C);
end

== matlab function pcc_backstepping_model_unaware_full_system_PID/Control/Full-system model-unaware PID/Map Delta f_p to pistons ==
  data: Delta_f_p input; f_p output; tol_q_stable input; mu_p_t0 input; b_C input; d_C input; l_p input; A_p input
function f_p = map_delta_fp_to_pistons(Delta_f_p, tol_q_stable, mu_p_t0, b_C, d_C, l_p, A_p)
    q_t0 = zeros(length(Delta_f_p), 1); % should be n_p x 1

    % introduce tolerance for numerical stability
    q_t0_stable = set_min_abs_val(q_t0, tol_q_stable);

    % potential forces by fluid
    G_p_mu_t0 = G_p_mu_fun(q_t0_stable, mu_p_t0, l_p, A_p, b_C, d_C);

    f_p = zeros(length(mu_p_t0), 1);
    for i=1:length(q_t0)
        f_p(2*i-1) = G_p_mu_t0(2*i-1) + 0.5*Delta_f_p(i);
        f_p(2*i) = G_p_mu_t0(2*i) - 0.5*Delta_f_p(i);
    end
end

== matlab function pcc_backstepping_model_unaware_full_system_PID/Control/Backstepping/Backstepping ==
  data: Gamma output; Pi output; q input; qdot input; q_ref input; tol_q_stable input; mu_p input; mu_p_dot input; Psi output; mu_p_t0 input; alpha input; l_p input; A_p input; m_p input; b_C input; d_C input; g input; k input; d input; d_p input; k_1 input; k_2 input
function [Gamma, Pi, Psi]= Psi_fun(q, qdot, q_ref, tol_q_stable, mu_p, ... 
                                   mu_p_dot, mu_p_t0, alpha, ...
                                   l_p, A_p, m_p, b_C, d_C, g, k, d, d_p, ...
                                   k_1, k_2)
    % introduce tolerance for numerical stability
    q_stable = set_min_abs_val(q, tol_q_stable);
                               
    % Proportional gain for approaching the desired piston position
    K_1 = diag(k_1);
    % Proportional gain for approaching the desired piston velocity
    K_2 = diag(k_2);
    
    % mass matrix of piston system
    M_p = diag(m_p);
    
    % Components of equations of motion
    B = B_fun(q_stable);
    B_dot = B_dot_fun(q_stable, qdot);
    C = C_fun(q_stable, qdot);
    G = G_fun(q_stable, alpha, g);
    
    % potential forces by fluid
    G_p_q = G_p_q_fun(q_stable, mu_p, l_p, A_p, b_C, d_C);
    G_p_mu = G_p_mu_fun(q_stable, mu_p, l_p, A_p, b_C, d_C);
    
    % acceleration of system
    qddot = -B^(-1)*(C*qdot + G + k.*q + d.*qdot + G_p_q);
    
    % Lyapunov function H
    dH_spc_dqdot = dH_spc_dqdot_fun(q_stable, qdot, alpha);
    dH_spc_dqdot_dot = dH_spc_dqdot_dot_fun(q_stable, qdot, qddot);

    % Gamma
    Gamma = Gamma_fun(q_stable, q_ref, mu_p_t0, alpha, l_p, A_p, b_C, d_C, g, k);
    dGamma_dq = dGamma_dq_fun(q_stable, q_ref, mu_p_t0, alpha, l_p, A_p, b_C, d_C, g, k);
    Gamma_dot = Gamma_dot_fun(q_stable, qdot, q_ref, mu_p_t0, alpha, l_p, A_p, b_C, d_C, g, k);
    dGamma_dot_dq = dGamma_dot_dq_fun(q_stable, qdot, q_ref, mu_p_t0, alpha, l_p, A_p, b_C, d_C, g, k);
    
    % Lemma 
    S = S_fun(q_stable, q_ref, mu_p, mu_p_t0, alpha, l_p, A_p, b_C, d_C, g, k);
    S_dot = S_dot_fun(q_stable, qdot, q_ref, mu_p, mu_p_t0, alpha, l_p, A_p, b_C, d_C, g, k);
    
    Pi = Gamma_dot - K_1*(mu_p - Gamma) + S'*(B^(-1))'*dH_spc_dqdot';
    
    Pi_dot = dGamma_dot_dq*qdot + dGamma_dq*qddot ...
             + K_1*dGamma_dq*qdot ...
             + S_dot'*(B^(-1))'*dH_spc_dqdot' ...
             - S'*(B^(-1)*B_dot*B^(-1))'*dH_spc_dqdot' ...
             + S'*(B^(-1))'*dH_spc_dqdot_dot;
    
    Psi = G_p_mu + M_p * Pi_dot - K_2*(mu_p_dot-Pi) - (mu_p-Gamma) + d_p.*Pi;
end

== matlab function pcc_backstepping_model_unaware_full_system_PID/Forward Kinematics ==
  data: alpha input; l input; x0 output; q input; x1 output; x2 output
function [x0, x1, x2] = forward_kinematics(alpha, l, q)
    % introduce tolerance for numerical stability
    q = set_min_abs_val(q, 0.005);

    x0 = q2x0_fun(l(1), q, alpha);
    x1 = q2x1_fun(l(2), q, alpha);
    x2 = q2x2_fun(l(3), q, alpha);
end

== matlab function pcc_backstepping_model_unaware_full_system_PID/Plant/PCC forward dynamics ==
  data: q input; qdot input; B input; qddot output; C input; G input; k input; d input; tau input; G_p_q input
function qddot  = pcc_forward_dynamics(q, qdot, B, C, G, k, d, tau, G_p_q)
   qddot = B^(-1)*(-(C*qdot)-G-(k.*q)-(d.*qdot)-G_p_q+tau);
end

== matlab function pcc_backstepping_model_unaware_full_system_PID/Initialisation/kapp2q ==
  data: kappa input; q output; l input
function q = kappa2q(kappa, l)
    q = [kappa(1) * l(1);
         kappa(2) * l(2);
         kappa(3) * l(3)];
end

== matlab function pcc_backstepping_model_unaware_full_system_PID/Plant/PCC Equations of Motion ==
  data: q input; qdot input; tol_q_stable input; alpha input; B output; g input; C output; G output
function [B, C, G]  = pcc_eom(q, qdot, tol_q_stable, alpha, g)
    % introduce tolerance for numerical stability
    q_stable = set_min_abs_val(q, tol_q_stable);
    
    B = B_fun(q_stable);
    
    C = C_fun(q_stable, qdot);
    
    G = G_fun(q_stable, alpha, g);
end

== matlab function pcc_backstepping_model_unaware_full_system_PID/Control/Inverse Dynamics Controller ==
  data: qddot_ref input; q input; tau_ref output; qdot input; B input; C input; G input; k input; d input
function tau_ref = fcn(qddot_ref, q, qdot, B, C, G, k, d)
    tau_ref = B*qddot_ref + C*qdot + G + k.*q + d.*qdot;
end
